simulink model "SSModelHeavy"  (R2016b)
settings: Solver=VariableStepAuto  StartTime=0.0  StopTime=5  RelTol=1e-3
values from neighbouring files (symbols this model uses):
  AH = [ 0 1 0 ... (first row only)    [CubeEdgeHeavy.m]
  BH = [ 0 ... (first row only)    [CubeEdgeHeavy.m]
  CH = eye(3)    [CubeEdgeHeavy.m]
  DH = zeros(3,1)    [CubeEdgeHeavy.m]
  KH = place(AH,BH,PH)    [CubeEdgeHeavy.m]
settings Model: Creator=Will  LastModifiedBy=Will
settings DataIOCC: Refine=5

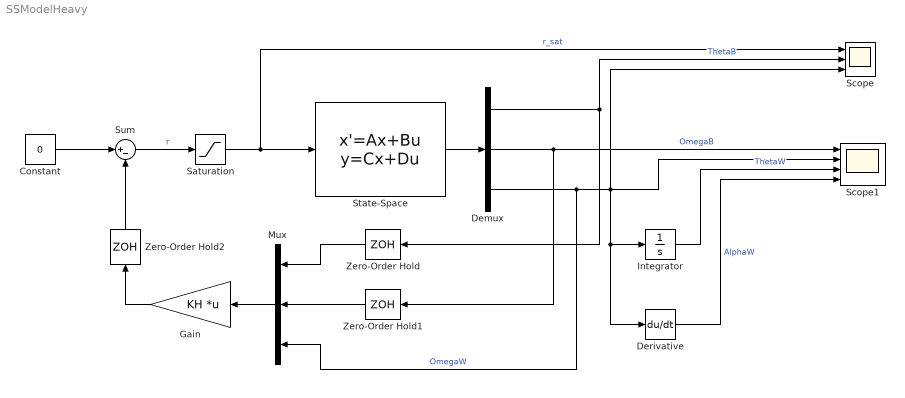
== system SSModelHeavy ==
  Constant : Constant  Value=0
  Demux : Demux  Outputs=3
  Derivative : Derivative
  Gain : Gain  Gain=KH  Multiplication=Matrix(K*u)
  Integrator : Integrator
  Mux : Mux  Inputs=3
  Saturation : Saturate  UpperLimit=6  LowerLimit=-6
  Scope : Scope  NumInputPorts=3
  Scope1 : Scope  NumInputPorts=4
  State-Space : StateSpace  A=AH  B=BH  C=CH  D=DH  X0=[.08 0 0]  ContinuousStateAttributes={'ThetaB', 'OmegaB', 'OmegaW'}
  Sum : Sum  Inputs=|+-
  Zero-Order Hold : ZeroOrderHold  SampleTime=1/100
  Zero-Order Hold1 : ZeroOrderHold  SampleTime=1/100
  Zero-Order Hold2 : ZeroOrderHold  SampleTime=.005
  wires:
  Demux/1 -> Scope/2, Zero-Order Hold/1  "ThetaB"
  Demux/2 -> Scope1/1, Zero-Order Hold1/1  "OmegaB"
  Demux/3 -> Mux/3, Scope/3, Scope1/2, Derivative/1, Integrator/1  "OmegaW"
  Sum/1 -> Saturation/1  "r"
  Constant/1 -> Sum/1
  State-Space/1 -> Demux/1
  Integrator/1 -> Scope1/3  "ThetaW"
  Derivative/1 -> Scope1/4  "AlphaW"
  Saturation/1 -> Scope/1, State-Space/1  "r_sat"
  Gain/1 -> Zero-Order Hold2/1
  Mux/1 -> Gain/1
  Zero-Order Hold/1 -> Mux/1
  Zero-Order Hold1/1 -> Mux/2
  Zero-Order Hold2/1 -> Sum/2
